simulink model "motor_interface"  (R2022b)
settings: Solver=FixedStepAuto  StartTime=0.0  StopTime=10.0  FixedStep=1e-3  RelTol=1e-3
libraries: motor_interface_lib x1
settings Model: Creator=dr_pa  LastModifiedBy=dr_pa
settings DataIOCC: ExternalInput=MI1.getElement('GOV_e_miCmd'),MI1.getElement('ptCAN_AMK_ActualValues1_Right'),MI1.getElement('ptCAN_AMK_ActualValues2_Right'),MI1.getElement('VD_n_RightMotorSpeedRequest'),MI1.getElement('VD_T_RightMotorTorqueLimitPositive'),MI1.getElement('VD_T_RightMotorTorqueLimitNegative'),MI1.getElement('ptCAN_AMK_ActualValues1_Left'),MI1.getElement('ptCAN_AMK_ActualValues2_Left'),MI1.getElement('VD_n_LeftMotorSpeedRequest'),MI1.getElement('VD_T_LeftMotorTorqueLimitPositive'),MI1.getElement('VD_T_LeftMotorTorqueLimitNegative')  LoadExternalInput=on

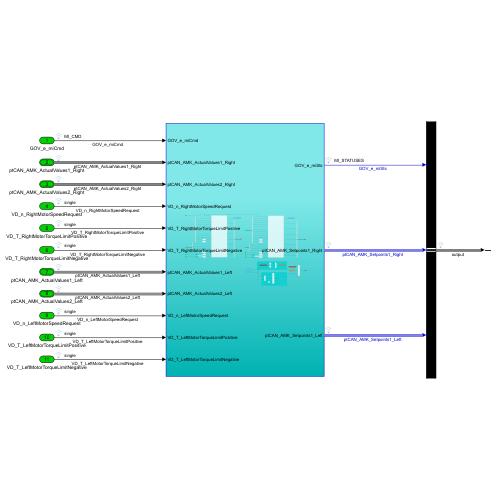
[thumbnail: Simulink's stored preview of the top-level diagram]
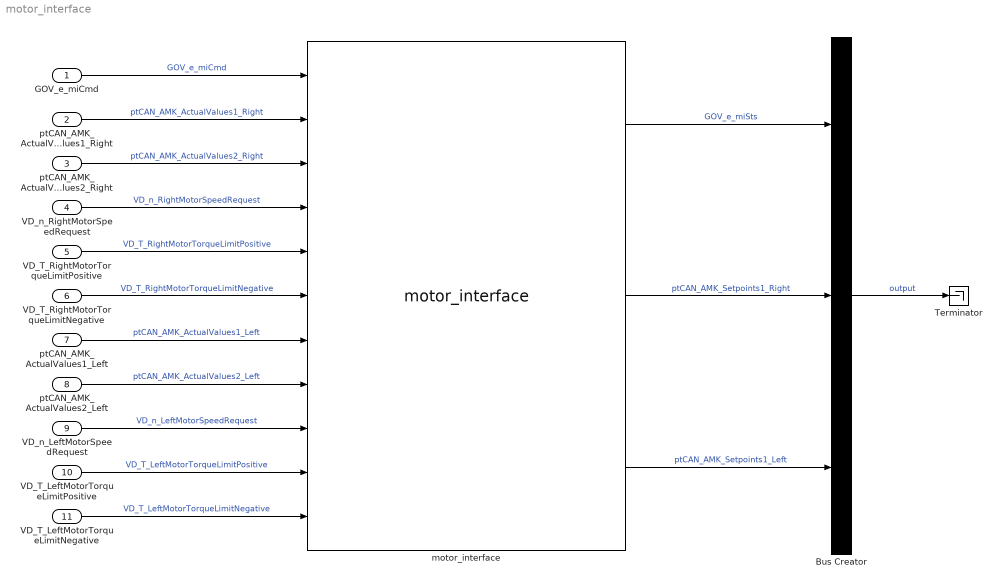
== system motor_interface ==
  GOV_e_miCmd : Inport  Interpolate=off
  ptCAN_AMK_ActualValues1_Right : Inport  Port=2  OutDataTypeStr=Bus: ptCAN_AMK_ActualValues1_Right_bus
  ptCAN_AMK_ActualValues2_Right : Inport  Port=3  OutDataTypeStr=Bus: ptCAN_AMK_ActualValues2_Right_bus
  VD_n_RightMotorSpeedRequest : Inport  Port=4  OutDataTypeStr=single
  VD_T_RightMotorTorqueLimitPositive : Inport  Port=5  OutDataTypeStr=single
  VD_T_RightMotorTorqueLimitNegative : Inport  Port=6  OutDataTypeStr=single
  ptCAN_AMK_ActualValues1_Left : Inport  Port=7  OutDataTypeStr=Bus: ptCAN_AMK_ActualValues1_Left_bus
  ptCAN_AMK_ActualValues2_Left : Inport  Port=8  OutDataTypeStr=Bus: ptCAN_AMK_ActualValues2_Left_bus
  VD_n_LeftMotorSpeedRequest : Inport  Port=9  OutDataTypeStr=single
  VD_T_LeftMotorTorqueLimitPositive : Inport  Port=10  OutDataTypeStr=single
  VD_T_LeftMotorTorqueLimitNegative : Inport  Port=11  OutDataTypeStr=single
  Bus Creator : BusCreator  Inputs=3
  Terminator : Terminator
  motor_interface : motor_interface_lib/motor_interface  SystemSampleTime=-1  VariantActivationTime=update diagram  Latency=0  AutoFrameSizeCalculation=off
  wires:
  Bus Creator/1 -> Terminator/1  "output"
  motor_interface/1 -> Bus Creator/1  "GOV_e_miSts"
  motor_interface/3 -> Bus Creator/3  "ptCAN_AMK_Setpoints1_Left"
  motor_interface/2 -> Bus Creator/2  "ptCAN_AMK_Setpoints1_Right"
  GOV_e_miCmd/1 -> motor_interface/1  "GOV_e_miCmd"
  ptCAN_AMK_ActualValues1_Right/1 -> motor_interface/2  "ptCAN_AMK_ActualValues1_Right"
  ptCAN_AMK_ActualValues2_Right/1 -> motor_interface/3  "ptCAN_AMK_ActualValues2_Right"
  VD_n_RightMotorSpeedRequest/1 -> motor_interface/4  "VD_n_RightMotorSpeedRequest"
  VD_T_RightMotorTorqueLimitPositive/1 -> motor_interface/5  "VD_T_RightMotorTorqueLimitPositive"
  VD_T_RightMotorTorqueLimitNegative/1 -> motor_interface/6  "VD_T_RightMotorTorqueLimitNegative"
  VD_n_LeftMotorSpeedRequest/1 -> motor_interface/9  "VD_n_LeftMotorSpeedRequest"
  VD_T_LeftMotorTorqueLimitPositive/1 -> motor_interface/10  "VD_T_LeftMotorTorqueLimitPositive"
  VD_T_LeftMotorTorqueLimitNegative/1 -> motor_interface/11  "VD_T_LeftMotorTorqueLimitNegative"
  ptCAN_AMK_ActualValues2_Left/1 -> motor_interface/8  "ptCAN_AMK_ActualValues2_Left"
  ptCAN_AMK_ActualValues1_Left/1 -> motor_interface/7  "ptCAN_AMK_ActualValues1_Left"
